simulink model "STEP2"  (R2020b)
settings: Solver=FixedStepAuto  StartTime=0  StopTime=inf  FixedStep=1  RelTol=1e-3
settings Model: Creator=Fong  LastModifiedBy=Fong

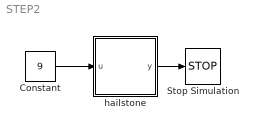
== system STEP2 ==
  Constant : Constant  Value=9
  Stop Simulation : Stop
  hailstone : Stateflow chart  TreatAsAtomicUnit=on
  wires:
  hailstone/1(y) -> Stop Simulation/1
  Constant/1 -> hailstone/1(u)

== stateflow chart STEP2/hailstone ==
  state Init
    entry:
    n2 = rem(n,2);
    y = false;
    exit:
    y = isequal(n,1);
  state Even
    entry,during:
    n = n/2;
    n2 = rem(n,2);
  state Odd
    entry,during:
    n = 3*(n-y)+1;
    n2 = rem(n,2);
  (default) -> Init : {n = u;}
  Init -> (junction 30) [order 1] : [n2 == 0]
  Init -> (junction 32) [order 2]
  (junction 30) -> Even
  (junction 32) -> Odd
  Odd -> Even : [n2 == 0]
  Even -> Odd : [n2 ~= 0]{y = isequal(n,1);}
  data: u input; n2 local double; y output; n local double
